simulink model "CaseD"  (R2016b)
settings: Solver=FixedStepAuto  StartTime=0.0  StopTime=time  FixedStep=dt  RelTol=1e-3
values from neighbouring files (symbols this model uses):
  C = [6; 0]    [main.m]
  dt = 0.01    [main.m]
  initial_eta = [1 0 0]'    [main.m]
  initial_eta_2 = [6 5 0]'    [main.m]
  initial_eta_4 = [7 0 0]'    [main.m]
  K_p = diag([0.2,0.2,0.1])    [main.m]
  mu = 0.1    [main.m]
  P_d = [2  0 ... (first row only)    [main.m]
  R = diag(r)    [main.m]
  r = [5; 3]    [main.m]
  U_max = 1    [main.m]
  U_ref = [(0:dt:time)' [zeros(floor(1*points/6),1) ... (first row only)    [main.m]
libraries: simulink x1
(part 2 of 2)

== matlab function CaseD/Line System 1-6/Update Law/Update Law ==
  data: U_s input; s_dot output; mu input; eta_d_s input; eta_d input; eta input
function s_dot = update(U_s, mu, eta_d_s, eta_d, eta)
diff = eta - eta_d;
diff(3) = angdiff(eta_d(3), eta(3)); % Order is important here
s_dot = U_s - mu/norm(eta_d_s) * -diff' * eta_d_s;

== matlab function CaseD/Line System 3-6/Control law1/MATLAB Function ==
  data: tau output; nu input; alpha_dot input; z_1 input
function tau = tau_function(nu, alpha_dot, z_1)
%% Parameters
% Rigid body and added mass
m = 14.79; 
I_z = 1.76; 
x_g = 0.0375; 
% y_g = 0.0;

X_u_dot = -2; 
Y_v_dot = -10; 
Y_r_dot = -0; 
N_r_dot = -1; 

% Max Values in Surge X, Sway Y and Yaw N
% X_max = 1.03; %[N]
% N_max = 2.50; %[N]
% Y_max = 0.98; %[N]

% Hydro surge, Hydro sway and Hydro Yaw Parameters
    % NB! We don't need most of them for now, that why they are commented
    % out, but don't remove them!!
X_u = -0.6555;  Y_v = -1.33;    N_v = 0.0; 
X_uu = 0.3545;  Y_vv = -2.776;  N_vv = -0.2088; 
X_uuu = -3.787; Y_vvv = -64.91; N_vvv = 0.0;
X_v = 0.0;      Y_r = -7.25;    N_r = -1.9; 
X_vv = -2.443;  Y_rr = -3.45;   N_rr = 0.75;
X_vvv = 0.0;    Y_rrr = 0.0;    N_rrr = 0.0;
                Y_rv = 0.805;   N_rv = 0.130;
                Y_vr = -0.845;  N_vr = 0.080;

%% Matrixes
u = nu(1); v = nu(2); r = nu(3); % I need a test values; 
    
a_11 = m-X_u_dot;   a_12 = 0;                   a_13 = 0; 
a_21 = 0;           a_22 = m-Y_v_dot ;          a_23 = m*x_g - Y_r_dot;
a_31 = 0;           a_32 = m*x_g - Y_r_dot;     a_33 = I_z - N_r_dot;

M = [a_11 a_12, a_13; a_12 a_22 a_23; a_31 a_32 a_33];

d_11_u =  -X_u - X_uu*abs(u) - X_uuu*u^2;
d_22_vr = -Y_v - Y_vv*abs(v) - Y_vvv*v^2   - Y_rv*abs(r);
d_23_vr = -Y_r - Y_vr*abs(v) - Y_rr*abs(r) - Y_rrr*r^2;
d_32_vr = -N_v - N_vv*abs(v) - N_vvv*v^2   - N_rv*abs(r);
d_33_vr = -N_r - N_vr*abs(v) - N_rr*abs(r) - N_rrr*r^2;

% The total damping matrix from the handbook page 53
D_tot = [d_11_u 0 0; 0 d_22_vr d_23_vr; 0 d_32_vr d_33_vr];

tau = D_tot*nu + M*alpha_dot - z_1;

== matlab function CaseD/Line System 3-6/Control law1/MATLAB Function1 ==
  data: eta input; z_1_dot output; eta_d input; eta_d_s input; nu input; s_dot input
function z_1_dot = derive_z_1(eta, eta_d, eta_d_s, nu, s_dot)
r = nu(3);
S = [0 -r 0; r 0 0; 0 0 0];

psi = eta(3);
R = [cos(psi) -sin(psi) 0;
     sin(psi) cos(psi)  0;
     0        0         1];
 
 z_1_a = eta - eta_d;
% Here is where our eta_d would jump because of the parametrization.
% Instead of doing something hacky, we can redefine the control
% law such that it has the exact same gain.
% To compute the angular difference, we use angdiff:
z_1_psi = angdiff(eta_d(3), eta(3));
z_1_a(3) = z_1_psi;
z_1 = R'*z_1_a;
z_1_dot = [0; 0; 0;];
z_1_dot = S'*z_1 + nu - R'*eta_d_s*s_dot;

== matlab function CaseD/Line System 2-6/Line Mapper/MATLAB Function ==
  data: s input; P_d input; s_proc_old input; eta_d output; eta_d_s output; s_proc output
function [eta_d, eta_d_s, s_proc] = linify(s, P_d, s_proc_old)
s = 1 - abs(mod(s, 2) - 1);
p_d = s.*[P_d(2, 1) - P_d(1, 1); P_d(2, 2) - P_d(1, 2)] + [P_d(1, 1); P_d(1, 2)];
psi_d = atan2(P_d(2, 2) - P_d(1, 2), P_d(2, 1) - P_d(1, 1));
if s_proc_old - s < 0
    psi_d = pi - psi_d;
end
p_d_s = [P_d(2, 1) - P_d(1, 1); P_d(2, 2) - P_d(1, 2)];
psi_d_s = 0;

eta_d = zeros(3, 1);
eta_d_s = zeros(3, 1);
eta_d = [p_d; psi_d];
eta_d_s = [p_d_s; psi_d_s];

s_proc = s;

== matlab function CaseD/Line System 2-6/Line Speed Gauge/Line ==
  data: U_ref input; U_s output; P_d input
function U_s = line(U_ref, P_d)
U_s = U_ref / sqrt(sum((P_d(:,2)-P_d(:,1)).^2));

== matlab function CaseD/Line System 3-6/Control law1/MATLAB Function2 ==
  data: eta_d input; eta input; z_1 output
function z_1 = compute_z_1(eta_d, eta)
psi = eta(3);
R = [cos(psi) -sin(psi) 0;
     sin(psi) cos(psi)  0;
     0        0         1];
z_1_a = eta - eta_d;
z_1_psi = angdiff(eta_d(3), eta(3));
z_1_a(3) = z_1_psi;
z_1 = R'*z_1_a;

== matlab function CaseD/Ellipse System 4-6/Control law1/MATLAB Function ==
  data: tau output; nu input; alpha_dot input; z_1 input
function tau = tau_function(nu, alpha_dot, z_1)
%% Parameters
% Rigid body and added mass
m = 14.79; 
I_z = 1.76; 
x_g = 0.0375; 
% y_g = 0.0;

X_u_dot = -2; 
Y_v_dot = -10; 
Y_r_dot = -0; 
N_r_dot = -1; 

% Max Values in Surge X, Sway Y and Yaw N
% X_max = 1.03; %[N]
% N_max = 2.50; %[N]
% Y_max = 0.98; %[N]

% Hydro surge, Hydro sway and Hydro Yaw Parameters
    % NB! We don't need most of them for now, that why they are commented
    % out, but don't remove them!!
X_u = -0.6555;  Y_v = -1.33;    N_v = 0.0; 
X_uu = 0.3545;  Y_vv = -2.776;  N_vv = -0.2088; 
X_uuu = -3.787; Y_vvv = -64.91; N_vvv = 0.0;
X_v = 0.0;      Y_r = -7.25;    N_r = -1.9; 
X_vv = -2.443;  Y_rr = -3.45;   N_rr = 0.75;
X_vvv = 0.0;    Y_rrr = 0.0;    N_rrr = 0.0;
                Y_rv = 0.805;   N_rv = 0.130;
                Y_vr = -0.845;  N_vr = 0.080;

%% Matrixes
u = nu(1); v = nu(2); r = nu(3); % I need a test values; 
    
a_11 = m-X_u_dot;   a_12 = 0;                   a_13 = 0; 
a_21 = 0;           a_22 = m-Y_v_dot ;          a_23 = m*x_g - Y_r_dot;
a_31 = 0;           a_32 = m*x_g - Y_r_dot;     a_33 = I_z - N_r_dot;

M = [a_11 a_12, a_13; a_12 a_22 a_23; a_31 a_32 a_33];

d_11_u =  -X_u - X_uu*abs(u) - X_uuu*u^2;
d_22_vr = -Y_v - Y_vv*abs(v) - Y_vvv*v^2   - Y_rv*abs(r);
d_23_vr = -Y_r - Y_vr*abs(v) - Y_rr*abs(r) - Y_rrr*r^2;
d_32_vr = -N_v - N_vv*abs(v) - N_vvv*v^2   - N_rv*abs(r);
d_33_vr = -N_r - N_vr*abs(v) - N_rr*abs(r) - N_rrr*r^2;

% The total damping matrix from the handbook page 53
D_tot = [d_11_u 0 0; 0 d_22_vr d_23_vr; 0 d_32_vr d_33_vr];

tau = D_tot*nu + M*alpha_dot - z_1;

== matlab function CaseD/Line System 3-6/Kinematic model/Rotation matrix ==
  data: psi input; R output
function R = rotation(psi)
R = [cos(psi) -sin(psi) 0;
     sin(psi) cos(psi)  0;
     0        0         1];

== matlab function CaseD/Line System 3-6/Line Mapper/MATLAB Function ==
  data: s input; s_proc_old input; eta_d output; eta_d_s output; P_d input; s_proc output
function [eta_d, eta_d_s, s_proc] = linify(s, s_proc_old, P_d)
s = 1 - abs(mod(s, 2) - 1);
p_d = s.*[P_d(2, 1) - P_d(1, 1); P_d(2, 2) - P_d(1, 2)] + [P_d(1, 1); P_d(1, 2)];
psi_d = atan2(P_d(2, 2) - P_d(1, 2), P_d(2, 1) - P_d(1, 1));
if s_proc_old - s < 0
    psi_d = pi - psi_d;
end
p_d_s = [P_d(2, 1) - P_d(1, 1); P_d(2, 2) - P_d(1, 2)];
psi_d_s = 0;

eta_d = zeros(3, 1);
eta_d_s = zeros(3, 1);
eta_d = [p_d; psi_d];
eta_d_s = [p_d_s; psi_d_s];

s_proc = s;

== matlab function CaseD/Line System 3-6/Line Speed Gauge/Line ==
  data: U_ref input; U_s output; P_d input
function U_s = line(U_ref, P_d)
U_s = U_ref / sqrt(sum((P_d(:,2)-P_d(:,1)).^2));

== matlab function CaseD/Line System 3-6/MATLAB Function ==
  data: scaled_U_max input; U_ref output; s input
function U_ref = variable_s(scaled_U_max, s)
s = 1 - abs(mod(s, 2) - 1);
U_ref = scaled_U_max*(1.01 + sin(2*pi*s - pi/2));

== matlab function CaseD/Line System 3-6/Update Law/Update Law ==
  data: U_s input; s_dot output; mu input; eta_d_s input; eta_d input; eta input
function s_dot = update(U_s, mu, eta_d_s, eta_d, eta)
s_dot = 0;
diff = eta - eta_d;
diff(3) = angdiff(eta_d(3), eta(3)); % Order is important here
s_dot = U_s - mu/norm(eta_d_s) * -diff' * eta_d_s;

== matlab function CaseD/Line System 1-6/Control law/MATLAB Function ==
  data: tau output; nu input; alpha_dot input; z_1 input
function tau = tau_function(nu, alpha_dot, z_1)
%% Parameters
% Rigid body and added mass
m = 14.79; 
I_z = 1.76; 
x_g = 0.0375; 
% y_g = 0.0;

X_u_dot = -2; 
Y_v_dot = -10; 
Y_r_dot = -0; 
N_r_dot = -1; 

% Max Values in Surge X, Sway Y and Yaw N
% X_max = 1.03; %[N]
% N_max = 2.50; %[N]
% Y_max = 0.98; %[N]

% Hydro surge, Hydro sway and Hydro Yaw Parameters
    % NB! We don't need most of them for now, that why they are commented
    % out, but don't remove them!!
X_u = -0.6555;  Y_v = -1.33;    N_v = 0.0; 
X_uu = 0.3545;  Y_vv = -2.776;  N_vv = -0.2088; 
X_uuu = -3.787; Y_vvv = -64.91; N_vvv = 0.0;
X_v = 0.0;      Y_r = -7.25;    N_r = -1.9; 
X_vv = -2.443;  Y_rr = -3.45;   N_rr = 0.75;
X_vvv = 0.0;    Y_rrr = 0.0;    N_rrr = 0.0;
                Y_rv = 0.805;   N_rv = 0.130;
                Y_vr = -0.845;  N_vr = 0.080;

%% Matrixes
u = nu(1); v = nu(2); r = nu(3); % I need a test values; 
    
a_11 = m-X_u_dot;   a_12 = 0;                   a_13 = 0; 
a_21 = 0;           a_22 = m-Y_v_dot ;          a_23 = m*x_g - Y_r_dot;
a_31 = 0;           a_32 = m*x_g - Y_r_dot;     a_33 = I_z - N_r_dot;

M = [a_11 a_12, a_13; a_12 a_22 a_23; a_31 a_32 a_33];

d_11_u =  -X_u - X_uu*abs(u) - X_uuu*u^2;
d_22_vr = -Y_v - Y_vv*abs(v) - Y_vvv*v^2   - Y_rv*abs(r);
d_23_vr = -Y_r - Y_vr*abs(v) - Y_rr*abs(r) - Y_rrr*r^2;
d_32_vr = -N_v - N_vv*abs(v) - N_vvv*v^2   - N_rv*abs(r);
d_33_vr = -N_r - N_vr*abs(v) - N_rr*abs(r) - N_rrr*r^2;

% The total damping matrix from the handbook page 53
D_tot = [d_11_u 0 0; 0 d_22_vr d_23_vr; 0 d_32_vr d_33_vr];

tau = D_tot*nu + M*alpha_dot - z_1;

== matlab function CaseD/Line System 1-6/Control law/MATLAB Function1 ==
  data: eta input; z_1_dot output; eta_d input; eta_d_s input; nu input; s_dot input
function z_1_dot = derive_z_1(eta, eta_d, eta_d_s, nu, s_dot)
r = nu(3);
S = [0 -r 0; r 0 0; 0 0 0];

psi = eta(3);
R = [cos(psi) -sin(psi) 0;
     sin(psi) cos(psi)  0;
     0        0         1];
 
 z_1_a = eta - eta_d;
% Here is where our eta_d would jump because of the parametrization.
% Instead of doing something hacky, we can redefine the control
% law such that it has the exact same gain.
% To compute the angular difference, we use angdiff:
z_1_psi = angdiff(eta_d(3), eta(3));
z_1_a(3) = z_1_psi;
z_1 = R'*z_1_a;
z_1_dot = S'*z_1 + nu - R'*eta_d_s*s_dot;

== matlab function CaseD/Line System 1-6/Control law/MATLAB Function2 ==
  data: eta_d input; eta input; z_1 output
function z_1 = compute_z_1(eta_d, eta)
psi = eta(3);
R = [cos(psi) -sin(psi) 0;
     sin(psi) cos(psi)  0;
     0        0         1];
z_1_a = eta - eta_d;
z_1_psi = angdiff(eta_d(3), eta(3));
z_1_a(3) = z_1_psi;
z_1 = R'*z_1_a;

== matlab function CaseD/Line System 1-6/Control law/MATLAB Function3 ==
  data: alpha_1 output; K_p input; eta input; eta_d input; eta_d_s input; U_s input
function alpha_1 = compute_alpha_1(K_p, eta, eta_d, eta_d_s, U_s)
psi = eta(3);
R = [cos(psi) -sin(psi) 0;
     sin(psi) cos(psi)  0;
     0        0         1];
 
z_1_a = eta - eta_d;
z_1_psi = angdiff(eta_d(3), eta(3));
z_1_a(3) = z_1_psi;
z_1 = R'*z_1_a;
alpha_1 = -K_p*z_1 + R'*eta_d_s*U_s;

== matlab function CaseD/Line System 1-6/Control law/MATLAB Function4 ==
  data: K_p input; z_1_dot input; eta input; eta_d_s input; nu input; U_s input; alpha_1_dot output; U_s_s input; eta_d_ss input; s_dot input
function alpha_1_dot = compute_alpha_1_dot(K_p, z_1_dot, eta, eta_d_s, nu, U_s, U_s_s, eta_d_ss, s_dot)
r = nu(3);
S = [0 -r 0; r 0 0; 0 0 0];
psi = eta(3);
R = [cos(psi) -sin(psi) 0;
     sin(psi) cos(psi)  0;
     0        0         1];

alpha_1_dot = -K_p*z_1_dot + S'*R'*eta_d_s*U_s + R'*eta_d_ss*s_dot*U_s + R'*eta_d_s*U_s_s*s_dot;

== matlab function CaseD/Line System 2-6/Control law1/MATLAB Function2 ==
  data: eta_d input; eta input; z_1 output
function z_1 = compute_z_1(eta_d, eta)
psi = eta(3);
R = [cos(psi) -sin(psi) 0;
     sin(psi) cos(psi)  0;
     0        0         1];
z_1_a = eta - eta_d;
z_1_psi = angdiff(eta_d(3), eta(3));
z_1_a(3) = z_1_psi;
z_1 = R'*z_1_a;

== matlab function CaseD/Line System 2-6/Control law1/MATLAB Function3 ==
  data: alpha_1 output; K_p input; eta input; eta_d input; eta_d_s input; U_s input
function alpha_1 = compute_alpha_1(K_p, eta, eta_d, eta_d_s, U_s)
psi = eta(3);
R = [cos(psi) -sin(psi) 0;
     sin(psi) cos(psi)  0;
     0        0         1];
 
z_1_a = eta - eta_d;
z_1_psi = angdiff(eta_d(3), eta(3));
z_1_a(3) = z_1_psi;
z_1 = R'*z_1_a;
alpha_1 = -K_p*z_1 + R'*eta_d_s*U_s;

== matlab function CaseD/Line System 2-6/Control law1/MATLAB Function4 ==
  data: K_p input; z_1_dot input; eta input; eta_d_s input; nu input; U_s input; alpha_1_dot output; U_s_s input; eta_d_ss input; s_dot input
function alpha_1_dot = compute_alpha_1_dot(K_p, z_1_dot, eta, eta_d_s, nu, U_s, U_s_s, eta_d_ss, s_dot)
r = nu(3);
S = [0 -r 0; r 0 0; 0 0 0];
psi = eta(3);
R = [cos(psi) -sin(psi) 0;
     sin(psi) cos(psi)  0;
     0        0         1];

alpha_1_dot = -K_p*z_1_dot + S'*R'*eta_d_s*U_s + R'*eta_d_ss*s_dot*U_s + R'*eta_d_s*U_s_s*s_dot;

== matlab function CaseD/Line System 2-6/Control law1/kinetics ==
  data: tau input; nu_dot output; nu input
function nu_dot = CSE1_nu_dot(tau,nu)

u   = nu(1);
v   = nu(2);
r   = nu(3);

tau = [tau(1);tau(2);tau(3)];
%% MATRICES

m    = 14.79;   I_z  =  1.7600;   x_g = 0.0375;       % x_g  =  0.0460; % Table B.1


%% Added mass
X_ud  =     -2.0;											% Table B.1
					Y_vd =     -1.0;	N_vd =    -0.0;		% Table B.1 guestimate
					Y_rd =      -0.0;	N_rd =    -1.0;		% Table B.1

%% Total mass matrix
m_11 = m-X_ud;
m_22 = m-Y_vd;
m_23 = m*x_g-Y_rd;
m_32 = m*x_g-N_vd;
m_33 = I_z-N_rd;

M    = [m_11 0    0
        0    m_22 m_23
        0    m_32 m_33];
	
%% Damping coefficients
% Comments at the end of the lines indicate the old values used.
X_u		= -0.6555;		X_v		= 0;
X_uu 	= 0.3545;		X_vv	= -2.443;
X_uuu 	= -3.787;		X_vvv	= 0;

						Y_v		= -1.33; 			Y_r		= -7.250; % Y_r
						Y_vv	= -2.776;			Y_rr	= -3.450; % Y_rr
						Y_vvv	= -64.91;			Y_rrr	= 0;
						
						Y_rv	= -0.805;			Y_vr	= -0.845; % Y_rv, Y_vr

						N_v		= 0;				N_r		= -1.900; % N_r
						N_vv	= -0.2088;			N_rr	= -0.750; % N_rr
						N_vvv	= 0;				N_rrr	= 0;
						
						N_rv	= 0.130;			N_vr	= 0.080; % N_rv, N_vr

%% Correolis matrix
c_13 = -(m-Y_vd)*v-(m*x_g-Y_rd)*r;
c_23 = (m-X_ud)*u;
C    = [0     0     c_13
        0     0     c_23
        -c_13 -c_23 0   ];

%% Assembly of the damping matrix
d_11 = -X_u - X_uu*u - X_uuu*u^2;
d_22 = -Y_v - Y_vv*v - Y_vvv*v^2 - Y_rv*abs(r);
d_33 = -N_r - N_rr*abs(r) - N_rrr*r^2 - N_vr*abs(v); % using abs(r)

d_12 = -X_v - X_vv*v - X_vvv*v^2;
d_23 = -Y_r - Y_rr*abs(r) - Y_rrr*r^2 - Y_vr*abs(v);
d_32 = -N_v - N_vv*v - N_vvv*v^2 - N_rv*abs(r);

D    = [d_11 d_12 0
        0    d_22 d_23
        0    d_32 d_33];



%% CALCULATION
nu_dot = M\(tau-(C+D)*nu);

== matlab function CaseD/Line System 2-6/Kinematic model1/Rotation matrix ==
  data: psi input; R output
function R = rotation(psi)
R = [cos(psi) -sin(psi) 0;
     sin(psi) cos(psi)  0;
     0        0         1];

== matlab function CaseD/Line System 3-6/Control law1/MATLAB Function3 ==
  data: alpha_1 output; K_p input; eta input; eta_d input; eta_d_s input; U_s input
function alpha_1 = compute_alpha_1(K_p, eta, eta_d, eta_d_s, U_s)
psi = eta(3);
R = [cos(psi) -sin(psi) 0;
     sin(psi) cos(psi)  0;
     0        0         1];
 
z_1_a = eta - eta_d;
z_1_psi = angdiff(eta_d(3), eta(3));
z_1_a(3) = z_1_psi;
z_1 = R'*z_1_a;
alpha_1 = -K_p*z_1 + R'*eta_d_s*U_s;

== matlab function CaseD/Line System 3-6/Control law1/MATLAB Function4 ==
  data: K_p input; z_1_dot input; eta input; eta_d_s input; nu input; U_s input; alpha_1_dot output; U_s_s input; eta_d_ss input; s_dot input
function alpha_1_dot = compute_alpha_1_dot(K_p, z_1_dot, eta, eta_d_s, nu, U_s, U_s_s, eta_d_ss, s_dot)
r = nu(3);
S = [0 -r 0; r 0 0; 0 0 0];
psi = eta(3);
R = [cos(psi) -sin(psi) 0;
     sin(psi) cos(psi)  0;
     0        0         1];

alpha_1_dot = -K_p*z_1_dot + S'*R'*eta_d_s*U_s + R'*eta_d_ss*s_dot*U_s + R'*eta_d_s*U_s_s*s_dot;

== matlab function CaseD/Line System 2-6/Update Law1/Update Law ==
  data: U_s input; s_dot output; mu input; eta_d_s input; eta_d input; eta input
function s_dot = update(U_s, mu, eta_d_s, eta_d, eta)
diff = eta - eta_d;
diff(3) = angdiff(eta_d(3), eta(3)); % Order is important here
s_dot = U_s - mu/norm(eta_d_s) * -diff' * eta_d_s;

== matlab function CaseD/Line System 3-6/Control law1/kinetics ==
  data: tau input; nu_dot output; nu input
function nu_dot = CSE1_nu_dot(tau,nu)

u   = nu(1);
v   = nu(2);
r   = nu(3);

tau = [tau(1);tau(2);tau(3)];
%% MATRICES

m    = 14.79;   I_z  =  1.7600;   x_g = 0.0375;       % x_g  =  0.0460; % Table B.1


%% Added mass
X_ud  =     -2.0;											% Table B.1
					Y_vd =     -1.0;	N_vd =    -0.0;		% Table B.1 guestimate
					Y_rd =      -0.0;	N_rd =    -1.0;		% Table B.1

%% Total mass matrix
m_11 = m-X_ud;
m_22 = m-Y_vd;
m_23 = m*x_g-Y_rd;
m_32 = m*x_g-N_vd;
m_33 = I_z-N_rd;

M    = [m_11 0    0
        0    m_22 m_23
        0    m_32 m_33];
	
%% Damping coefficients
% Comments at the end of the lines indicate the old values used.
X_u		= -0.6555;		X_v		= 0;
X_uu 	= 0.3545;		X_vv	= -2.443;
X_uuu 	= -3.787;		X_vvv	= 0;

						Y_v		= -1.33; 			Y_r		= -7.250; % Y_r
						Y_vv	= -2.776;			Y_rr	= -3.450; % Y_rr
						Y_vvv	= -64.91;			Y_rrr	= 0;
						
						Y_rv	= -0.805;			Y_vr	= -0.845; % Y_rv, Y_vr

						N_v		= 0;				N_r		= -1.900; % N_r
						N_vv	= -0.2088;			N_rr	= -0.750; % N_rr
						N_vvv	= 0;				N_rrr	= 0;
						
						N_rv	= 0.130;			N_vr	= 0.080; % N_rv, N_vr

%% Correolis matrix
c_13 = -(m-Y_vd)*v-(m*x_g-Y_rd)*r;
c_23 = (m-X_ud)*u;
C    = [0     0     c_13
        0     0     c_23
        -c_13 -c_23 0   ];

%% Assembly of the damping matrix
d_11 = -X_u - X_uu*u - X_uuu*u^2;
d_22 = -Y_v - Y_vv*v - Y_vvv*v^2 - Y_rv*abs(r);
d_33 = -N_r - N_rr*abs(r) - N_rrr*r^2 - N_vr*abs(v); % using abs(r)

d_12 = -X_v - X_vv*v - X_vvv*v^2;
d_23 = -Y_r - Y_rr*abs(r) - Y_rrr*r^2 - Y_vr*abs(v);
d_32 = -N_v - N_vv*v - N_vvv*v^2 - N_rv*abs(r);

D    = [d_11 d_12 0
        0    d_22 d_23
        0    d_32 d_33];



%% CALCULATION
nu_dot = M\(tau-(C+D)*nu);

== matlab function CaseD/Ellipse System 4-6/Control law1/MATLAB Function1 ==
  data: eta input; z_1_dot output; eta_d input; eta_d_s input; nu input; s_dot input
function z_1_dot = derive_z_1(eta, eta_d, eta_d_s, nu, s_dot)
r = nu(3);
S = [0 -r 0; r 0 0; 0 0 0];

psi = eta(3);
R = [cos(psi) -sin(psi) 0;
     sin(psi) cos(psi)  0;
     0        0         1];
 
 z_1_a = eta - eta_d;
% Here is where our eta_d would jump because of the parametrization.
% Instead of doing something hacky, we can redefine the control
% law such that it has the exact same gain.
% To compute the angular difference, we use angdiff:
z_1_psi = angdiff(eta_d(3), eta(3));
z_1_a(3) = z_1_psi;
z_1 = R'*z_1_a;
z_1_dot = S'*z_1 + nu - R'*eta_d_s*s_dot;
z_1_dot = [0 0 0]';

== matlab function CaseD/Ellipse System 4-6/Control law1/MATLAB Function2 ==
  data: eta_d input; eta input; z_1 output
function z_1 = compute_z_1(eta_d, eta)
psi = eta(3);
R = [cos(psi) -sin(psi) 0;
     sin(psi) cos(psi)  0;
     0        0         1];
z_1_a = eta - eta_d;
z_1_psi = angdiff(eta_d(3), eta(3));
z_1_a(3) = z_1_psi;
z_1 = R'*z_1_a;

== matlab function CaseD/Ellipse System 4-6/Control law1/MATLAB Function3 ==
  data: alpha_1 output; K_p input; eta input; eta_d input; eta_d_s input; U_s input
function alpha_1 = compute_alpha_1(K_p, eta, eta_d, eta_d_s, U_s)
psi = eta(3);
R = [cos(psi) -sin(psi) 0;
     sin(psi) cos(psi)  0;
     0        0         1];
 
z_1_a = eta - eta_d;
z_1_psi = angdiff(eta_d(3), eta(3));
z_1_a(3) = z_1_psi;
z_1 = R'*z_1_a;
alpha_1 = -K_p*z_1 + R'*eta_d_s*U_s;

== matlab function CaseD/Ellipse System 4-6/Control law1/MATLAB Function4 ==
  data: K_p input; z_1_dot input; eta input; eta_d_s input; nu input; U_s input; alpha_1_dot output; U_s_s input; eta_d_ss input; s_dot input
function alpha_1_dot = compute_alpha_1_dot(K_p, z_1_dot, eta, eta_d_s, nu, U_s, U_s_s, eta_d_ss, s_dot)
r = nu(3);
S = [0 -r 0; r 0 0; 0 0 0];
psi = eta(3);
R = [cos(psi) -sin(psi) 0;
     sin(psi) cos(psi)  0;
     0        0         1];

alpha_1_dot = -K_p*z_1_dot + S'*R'*eta_d_s*U_s + R'*eta_d_ss*s_dot*U_s + R'*eta_d_s*U_s_s*s_dot;

== matlab function CaseD/Ellipse System 4-6/Control law1/kinetics ==
  data: tau input; nu_dot output; nu input
function nu_dot = CSE1_nu_dot(tau,nu)

u   = nu(1);
v   = nu(2);
r   = nu(3);

tau = [tau(1);tau(2);tau(3)];
%% MATRICES

m    = 14.79;   I_z  =  1.7600;   x_g = 0.0375;       % x_g  =  0.0460; % Table B.1


%% Added mass
X_ud  =     -2.0;											% Table B.1
					Y_vd =     -1.0;	N_vd =    -0.0;		% Table B.1 guestimate
					Y_rd =      -0.0;	N_rd =    -1.0;		% Table B.1

%% Total mass matrix
m_11 = m-X_ud;
m_22 = m-Y_vd;
m_23 = m*x_g-Y_rd;
m_32 = m*x_g-N_vd;
m_33 = I_z-N_rd;

M    = [m_11 0    0
        0    m_22 m_23
        0    m_32 m_33];
	
%% Damping coefficients
% Comments at the end of the lines indicate the old values used.
X_u		= -0.6555;		X_v		= 0;
X_uu 	= 0.3545;		X_vv	= -2.443;
X_uuu 	= -3.787;		X_vvv	= 0;

						Y_v		= -1.33; 			Y_r		= -7.250; % Y_r
						Y_vv	= -2.776;			Y_rr	= -3.450; % Y_rr
						Y_vvv	= -64.91;			Y_rrr	= 0;
						
						Y_rv	= -0.805;			Y_vr	= -0.845; % Y_rv, Y_vr

						N_v		= 0;				N_r		= -1.900; % N_r
						N_vv	= -0.2088;			N_rr	= -0.750; % N_rr
						N_vvv	= 0;				N_rrr	= 0;
						
						N_rv	= 0.130;			N_vr	= 0.080; % N_rv, N_vr

%% Correolis matrix
c_13 = -(m-Y_vd)*v-(m*x_g-Y_rd)*r;
c_23 = (m-X_ud)*u;
C    = [0     0     c_13
        0     0     c_23
        -c_13 -c_23 0   ];

%% Assembly of the damping matrix
d_11 = -X_u - X_uu*u - X_uuu*u^2;
d_22 = -Y_v - Y_vv*v - Y_vvv*v^2 - Y_rv*abs(r);
d_33 = -N_r - N_rr*abs(r) - N_rrr*r^2 - N_vr*abs(v); % using abs(r)

d_12 = -X_v - X_vv*v - X_vvv*v^2;
d_23 = -Y_r - Y_rr*abs(r) - Y_rrr*r^2 - Y_vr*abs(v);
d_32 = -N_v - N_vv*v - N_vvv*v^2 - N_rv*abs(r);

D    = [d_11 d_12 0
        0    d_22 d_23
        0    d_32 d_33];



%% CALCULATION
nu_dot = M\(tau-(C+D)*nu);
